simulink model "Variable_Mass_Station_Keeping"  (R2017b)
settings: Solver=VariableStepAuto  StartTime=0.0  StopTime=100  RelTol=1e-3
values from neighbouring files (symbols this model uses):
  A_define = A(1:12,1:12)    [F16_init.m]
  A_la_define = A_define([2,4,6,9,10,12],[2,4,6,9,10,12])    [Controller_para.m]
  A_lon_define = A_define([1,3,5,7,8,11],[1,3,5,7,8,11])    [Controller_para.m]
  airSpeed = 393.720000000000    (= 393.72)    [F16_init.m]
  alpha0 = trimAlpha*180/pi    (= 6.62393794015)    [F16_init.m]
  altitude = 9843    [F16_init.m]
  B_define = A(1:12,13:16)    [F16_init.m]
  B_la_define = B_define([2,4,6,9,10,12],3:4)    [Controller_para.m]
  B_lon_define = B_define([1,3,5,7,8,11],1:2)    [Controller_para.m]
  b_ref = 30.0    (= 30)    [F16_init.m]
  C_la = [1,0,zeros(1,4)]    [F16_init.m]
  C_lon = [1,0,zeros(1,4);0,1,zeros(1,4)]    [F16_init.m]
  CC_la = P_la * B_la_define    [Controller_para.m]
  CC_lon = P_lon * B_lon_define    [Controller_para.m]
  dLEF = 0    [F16_init.m]
  fi_flag = 1    [F16_init.m]
  Inertia = [9496,0,-982.0;0,55814.0,0;-982.0,0,63100.0]    [F16_init.m]
  Ki_la = -k_la(:,9)    [F16_init.m]
  Ki_lon = -k_lon(:,9:10)    [F16_init.m]
  kp_la = Kp_define(3:4,[2,4,6,9,10,12])    [Controller_para.m]    (also in F16_init.m)
  kp_lon = Kp_define(1:2,[1,3,5,7,8,11])    [Controller_para.m]    (also in F16_init.m)
  mass = 636.94    [F16_init.m]
  trim_ail = 0.00874607850103852    (= 0.00874607850104)    [F16_init.m]
  trim_control = [trim_thrust;trim_ele;trim_ail;trim_rud]    [F16_init.m]
  trim_ele = -2.97973164860638    (= -2.97973164861)    [F16_init.m]
  trim_rud = 0.0680302158182712    (= 0.0680302158183)    [F16_init.m]
  trim_state = [0;0;0;0;trimAlpha;0;airSpeed;trimAlpha;0;0;0;0]    [F16_init.m]
  trim_thrust = 2279.08519954656    (= 2279.08519955)    [F16_init.m]
  v_oil = 1.37    [F16_init.m]
undefined symbols (not defined in the file or in its folder): F, MIL
libraries: aerolibasang x8, aerolibconvert2 x8, aerolibobsolete x3, aerolibatmos2 x2, aerolibadyn x2, aerolibwind2 x1, shared6dof x1
(part 2 of 2)

== matlab function Variable_Mass_Station_Keeping/Constant Mass Model/Observer/Nonlinear Term ==
  data: trimed_states input; y output; A_la_define input; A_lon_define input; trim_states input
function y = fcn(trimed_states,A_la_define,A_lon_define,trim_states)
%% 原状态值（配平前的）
ori_states = trimed_states + trim_states;
phi_ori = ori_states(4);
theta_ori = ori_states(5);
psi_ori = ori_states(6);
Vr_ori = ori_states(7);
alpha_ori = ori_states(8);
beta_ori = ori_states(9);
p_ori = ori_states(10);
q_ori = ori_states(11);
r_ori = ori_states(12);

ug_ori = Vr_ori * cos(alpha_ori) * cos(beta_ori);
vg_ori = Vr_ori * sin(beta_ori);
wg_ori = Vr_ori * sin(alpha_ori) * cos(beta_ori);

xg_ori = ug_ori*cos(theta_ori)*cos(psi_ori) + vg_ori*(sin(phi_ori)*sin(theta_ori)*cos(psi_ori)-cos(phi_ori)*sin(psi_ori)) ...
     + wg_ori*(sin(phi_ori)*sin(psi_ori)+cos(phi_ori)*sin(theta_ori)*cos(psi_ori));
yg_ori = ug_ori*cos(theta_ori)*sin(psi_ori) + vg_ori*(sin(phi_ori)*sin(theta_ori)*sin(psi_ori)+cos(phi_ori)*cos(psi_ori)) ...
     + wg_ori*(-sin(phi_ori)*cos(psi_ori) + cos(phi_ori)*sin(theta_ori)*sin(psi_ori));
hg_ori = ug_ori*sin(theta_ori) - vg_ori*sin(phi_ori)*cos(theta_ori) - wg_ori*cos(phi_ori)*cos(theta_ori);
%% 差状态值（配平后的）
phi_trimed = trimed_states(4);
theta_trimed = trimed_states(5);
psi_trimed = trimed_states(6);
Vr_trimed = trimed_states(7);
alpha_trimed = trimed_states(8);
beta_trimed = trimed_states(9);
p_trimed = trimed_states(10);
q_trimed = trimed_states(11);
r_trimed = trimed_states(12);

% x_nonlinear = Vr_ori * cos(theta_ori - alpha_ori) - A_lon_define(1,3) * theta_trimed - Vr_ori;
% y_nonlinear = Vr_ori * cos(theta_ori - alpha_ori) * sin(psi_ori + beta_ori) - A_la_define(1,2) * phi_trimed - A_la_define(1,3) * psi_trimed - A_la_define(1,4) * beta_trimed;
% h_nonlinear = hg_ori  - A_lon_define(2,3) * (theta_trimed - alpha_trimed);

x_nonlinear = Vr_ori * cos(theta_ori - alpha_ori) - trim_states(7)*cos(trim_states(5)-trim_states(8)) - A_lon_define(1,3) * theta_trimed - Vr_trimed;
y_nonlinear = yg_ori - A_la_define(1,2) * phi_trimed - A_la_define(1,3) * psi_trimed - A_la_define(1,4) * beta_trimed;
h_nonlinear = Vr_ori * sin(theta_ori - alpha_ori) - A_lon_define(2,3) * (theta_trimed - alpha_trimed);
psi_nonlinear = (q_ori*sin(phi_ori) + r_ori*cos(phi_ori))/cos(theta_ori) - A_la_define(3,6) * r_trimed;  % psi
phi_nonlinear = p_ori + tan(theta_ori)*(q_ori*sin(phi_ori)+r_ori*cos(phi_ori)) - A_la_define(2,5) * p_trimed - A_la_define(2,6) * r_trimed;  % phi


y = [x_nonlinear; y_nonlinear; h_nonlinear; phi_nonlinear; 0; psi_nonlinear; 0;0;0;0;0;0];

== matlab function Variable_Mass_Station_Keeping/Constant Mass Model/pri_sys_controller/MATLAB Function ==
  settings: updateMethod=DISCRETE
  data: y output; t input
function y = fcn(t)

persistent tt;
if(isempty(tt))
  tt=0;
end

t1 = t-tt;
% if t1 < 10
%     xx = 0;
% elseif  t1 >= 10 && t1 < 70
%     xx = 50*sin(0.025*(t1-10));
% elseif  t1 >= 70 && t1 < 90
%     xx = 50;
% elseif  t1 >= 90 && t1 < 150
%     xx = 50-15*sin(0.025*(t1-90));
% else
%     xx = 35;
% end

% if t1 < 10
%     xx = 0;
% elseif  t1 >= 10 && t1 < 70
%     xx = 1*sin(0.025*(t1-10));
% else
%     xx = 1;
% end
xx = 0;

zz = 0;

y = [xx;zz];

end

== matlab function Variable_Mass_Station_Keeping/Variable Mass Model/sec_sys_controller/Lon_Controller ==
  data: s output; Sec_States input; output output; Pri_States input; A_lon_define input; B_lon_define input; CC_lon input; trim_states input
function [s,output] = Lon_Controller(Sec_States,Pri_States,A_lon_define,B_lon_define,CC_lon,trim_states)
Sec_lon = Sec_States([1,3,5,7,8,11]);  % 辅系统纵向通道状态
ori_states = Sec_States + Pri_States + trim_states;
theta_ori = ori_states(5);
Vr_ori = ori_states(7);
alpha_ori = ori_states(8);

trimed_states = Sec_States + Pri_States;
theta_trimed = trimed_states(5);
Vr_trimed = trimed_states(7);
alpha_trimed = trimed_states(8);

%%  辅系统非线性项g(x)
first_term = Vr_ori * cos(theta_ori - alpha_ori)  - trim_states(7)*cos(trim_states(5)-trim_states(8)) -  A_lon_define(1,3) * theta_trimed - Vr_trimed;
second_term = Vr_ori * sin(theta_ori - alpha_ori) - A_lon_define(2,3) * (theta_trimed - alpha_trimed);
NonLinear = [first_term;second_term;0;0;0;0];
% NonLinear = 0;
%% 滑模控制器结构
s = CC_lon' * Sec_lon;    % 定义滑模面
gain_lon = inv(CC_lon'*B_lon_define);
k1 = [1,0;0,1];
temp = CC_lon'* (A_lon_define * Sec_lon + NonLinear) + k1 * s;
output = -gain_lon * temp;
%% 反馈线性化控制器结构
% s = CC_lon' * Sec_lon;    % 定义输出函数 y = C * x
% gain_lon = inv(CC_lon'*B_lon_define);
% output = gain_lon * (-s - CC_lon' * NonLinear - CC_lon' * A_lon_define * Sec_lon);
end

== matlab function Variable_Mass_Station_Keeping/Variable Mass Model/sec_sys_controller/Lat_Controller ==
  data: Pri_States input; Sec_States input; output output; A_la_define input; B_la_define input; CC_la input; s output; trim_states input
function [output,s] = Lat_Controller(Pri_States,Sec_States,A_la_define,B_la_define,CC_la,trim_states)
Sec_lat = Sec_States([2,4,6,9,10,12]);  % 辅系统横侧向通道状态
ori_states = Sec_States + Pri_States + trim_states;
phi_ori = ori_states(4);
theta_ori = ori_states(5);
psi_ori = ori_states(6);
Vr_ori = ori_states(7);
alpha_ori = ori_states(8);
beta_ori = ori_states(9);
p_ori = ori_states(10);
q_ori = ori_states(11);
r_ori = ori_states(12);

ug_ori = Vr_ori * cos(alpha_ori) * cos(beta_ori);
vg_ori = Vr_ori * sin(beta_ori);
wg_ori = Vr_ori * sin(alpha_ori) * cos(beta_ori);

yg_ori = ug_ori*cos(theta_ori)*sin(psi_ori) + vg_ori*(sin(phi_ori)*sin(theta_ori)*sin(psi_ori)+cos(phi_ori)*cos(psi_ori)) ...
     + wg_ori*(-sin(phi_ori)*cos(psi_ori)+cos(phi_ori)*sin(theta_ori)*sin(psi_ori));
 
trimed_states = Sec_States + Pri_States;
phi_trimed = trimed_states(4);
theta_trimed = trimed_states(5);
psi_trimed = trimed_states(6);
Vr_trimed = trimed_states(7);
alpha_trimed = trimed_states(8);
beta_trimed = trimed_states(9);
p_trimed = trimed_states(10);
q_trimed = trimed_states(11);
r_trimed = trimed_states(12);
%%  辅系统非线性项g(x)
first_term = yg_ori - A_la_define(1,2) * phi_trimed - A_la_define(1,3) * psi_trimed - A_la_define(1,4) * beta_trimed;
% first_term = Vr_ori * cos(theta_ori - alpha_ori) * sin(psi_ori + beta_ori) - A_la_define(1,2) * phi_trimed - A_la_define(1,3) * psi_trimed - A_la_define(1,4) * beta_trimed;
second_term = p_ori + tan(theta_ori)*(q_ori*sin(phi_ori)+r_ori*cos(phi_ori)) - A_la_define(2,5) * p_trimed - A_la_define(2,6) * r_trimed;  % phi
third_term = (q_ori*sin(phi_ori) + r_ori*cos(phi_ori))/cos(theta_ori) - A_la_define(3,6) * r_trimed;  % psi
NonLinear = [first_term;second_term;third_term;0;0;0];
% NonLinear = 0;
%% 滑模控制器结构
s = CC_la' * Sec_lat;    % 定义滑模面
gain_lat = inv(CC_la'*B_la_define);
k1 = [1,0;0,1];
temp = CC_la'* (A_la_define * Sec_lat + NonLinear) + k1 * s ;
output = -gain_lat * temp;
%% 反馈线性化控制器结构
% s = CC_la' * Sec_lat;    % 定义输出函数 y = C * x
% gain_lat = inv(CC_la'*B_la_define);
% output = gain_lat * (-s - CC_la' * NonLinear - CC_la' * A_la_define * Sec_lat);
end

== matlab function Variable_Mass_Station_Keeping/Constant Mass Model/pri_sys_controller/MATLAB Function1 ==
  settings: updateMethod=DISCRETE
  data: y output; t input
function y = fcn(t)

persistent tt;
if(isempty(tt))
  tt=0;
end

t1 = t-tt;

% if t1 < 90
%     yy = 0;
% elseif  t1 >= 90 && t1 < 150
%     yy = 50*sin(0.025*(t1-90));
% else
%     yy = 50;
% end
% end

yy = 0;
y = yy;

== matlab function Variable_Mass_Station_Keeping/Constant Mass Model/pri_sys_controller/MATLAB Function3 ==
  data: u input; y output
function y = fcn(u)

y = u([1,3,5,7,8,11]);

== matlab function Variable_Mass_Station_Keeping/Variable Mass Model/pri_sys_controller/MATLAB Function1 ==
  settings: updateMethod=DISCRETE
  data: y output; t input
function y = fcn(t)

persistent tt;
if(isempty(tt))
  tt=0;
end

t1 = t-tt;

% if t1 < 90
%     yy = 0;
% elseif  t1 >= 90 && t1 < 150
%     yy = 50*sin(0.025*(t1-90));
% else
%     yy = 50;
% end

yy = 0;

y = yy;

end

== matlab function Variable_Mass_Station_Keeping/Variable Mass Model/Observer/Nonlinear Term ==
  data: trimed_states input; y output; A_la_define input; A_lon_define input; trim_states input
function y = fcn(trimed_states,A_la_define,A_lon_define,trim_states)
%% 原状态值（配平前的）
ori_states = trimed_states + trim_states;
phi_ori = ori_states(4);
theta_ori = ori_states(5);
psi_ori = ori_states(6);
Vr_ori = ori_states(7);
alpha_ori = ori_states(8);
beta_ori = ori_states(9);
p_ori = ori_states(10);
q_ori = ori_states(11);
r_ori = ori_states(12);

ug_ori = Vr_ori * cos(alpha_ori) * cos(beta_ori);
vg_ori = Vr_ori * sin(beta_ori);
wg_ori = Vr_ori * sin(alpha_ori) * cos(beta_ori);

xg_ori = ug_ori*cos(theta_ori)*cos(psi_ori) + vg_ori*(sin(phi_ori)*sin(theta_ori)*cos(psi_ori)-cos(phi_ori)*sin(psi_ori)) ...
     + wg_ori*(sin(phi_ori)*sin(psi_ori)+cos(phi_ori)*sin(theta_ori)*cos(psi_ori));
yg_ori = ug_ori*cos(theta_ori)*sin(psi_ori) + vg_ori*(sin(phi_ori)*sin(theta_ori)*sin(psi_ori)+cos(phi_ori)*cos(psi_ori)) ...
     + wg_ori*(-sin(phi_ori)*cos(psi_ori) + cos(phi_ori)*sin(theta_ori)*sin(psi_ori));
hg_ori = ug_ori*sin(theta_ori) - vg_ori*sin(phi_ori)*cos(theta_ori) - wg_ori*cos(phi_ori)*cos(theta_ori);
%% 差状态值（配平后的）
phi_trimed = trimed_states(4);
theta_trimed = trimed_states(5);
psi_trimed = trimed_states(6);
Vr_trimed = trimed_states(7);
alpha_trimed = trimed_states(8);
beta_trimed = trimed_states(9);
p_trimed = trimed_states(10);
q_trimed = trimed_states(11);
r_trimed = trimed_states(12);

% x_nonlinear = Vr_ori * cos(theta_ori - alpha_ori) - A_lon_define(1,3) * theta_trimed - Vr_ori;
% y_nonlinear = Vr_ori * cos(theta_ori - alpha_ori) * sin(psi_ori + beta_ori) - A_la_define(1,2) * phi_trimed - A_la_define(1,3) * psi_trimed - A_la_define(1,4) * beta_trimed;
% h_nonlinear = hg_ori  - A_lon_define(2,3) * (theta_trimed - alpha_trimed);

x_nonlinear = Vr_ori * cos(theta_ori - alpha_ori) - trim_states(7)*cos(trim_states(5)-trim_states(8)) - A_lon_define(1,3) * theta_trimed - Vr_trimed;
y_nonlinear = yg_ori - A_la_define(1,2) * phi_trimed - A_la_define(1,3) * psi_trimed - A_la_define(1,4) * beta_trimed;
h_nonlinear = Vr_ori * sin(theta_ori - alpha_ori) - A_lon_define(2,3) * (theta_trimed - alpha_trimed);
psi_nonlinear = (q_ori*sin(phi_ori) + r_ori*cos(phi_ori))/cos(theta_ori) - A_la_define(3,6) * r_trimed;  % psi
phi_nonlinear = p_ori + tan(theta_ori)*(q_ori*sin(phi_ori)+r_ori*cos(phi_ori)) - A_la_define(2,5) * p_trimed - A_la_define(2,6) * r_trimed;  % phi


y = [x_nonlinear; y_nonlinear; h_nonlinear; phi_nonlinear; 0; psi_nonlinear; 0;0;0;0;0;0];

== matlab function Variable_Mass_Station_Keeping/Constant Mass Model/pri_sys_controller/MATLAB Function4 ==
  data: u input; y output
function y = fcn(u)

y = u([2,4,6,9,10,12]);

== matlab function Variable_Mass_Station_Keeping/Variable Mass Model/pri_sys_controller/MATLAB Function3 ==
  data: u input; y output
function y = fcn(u)

y = u([1,3,5,7,8,11]);

== matlab function Variable_Mass_Station_Keeping/Variable Mass Model/pri_sys_controller/MATLAB Function4 ==
  data: u input; y output
function y = fcn(u)

y = u([2,4,6,9,10,12]);

== matlab function Variable_Mass_Station_Keeping/Constant Mass Model/sec_sys_controller/Lat_Controller ==
  data: Pri_States input; Sec_States input; output output; A_la_define input; B_la_define input; CC_la input; s output; trim_states input
function [output,s] = Lat_Controller(Pri_States,Sec_States,A_la_define,B_la_define,CC_la,trim_states)
Sec_lat = Sec_States([2,4,6,9,10,12]);  % 辅系统横侧向通道状态
ori_states = Sec_States + Pri_States + trim_states;
phi_ori = ori_states(4);
theta_ori = ori_states(5);
psi_ori = ori_states(6);
Vr_ori = ori_states(7);
alpha_ori = ori_states(8);
beta_ori = ori_states(9);
p_ori = ori_states(10);
q_ori = ori_states(11);
r_ori = ori_states(12);

ug_ori = Vr_ori * cos(alpha_ori) * cos(beta_ori);
vg_ori = Vr_ori * sin(beta_ori);
wg_ori = Vr_ori * sin(alpha_ori) * cos(beta_ori);

yg_ori = ug_ori*cos(theta_ori)*sin(psi_ori) + vg_ori*(sin(phi_ori)*sin(theta_ori)*sin(psi_ori)+cos(phi_ori)*cos(psi_ori)) ...
     + wg_ori*(-sin(phi_ori)*cos(psi_ori)+cos(phi_ori)*sin(theta_ori)*sin(psi_ori));
 
trimed_states = Sec_States + Pri_States;
phi_trimed = trimed_states(4);
theta_trimed = trimed_states(5);
psi_trimed = trimed_states(6);
Vr_trimed = trimed_states(7);
alpha_trimed = trimed_states(8);
beta_trimed = trimed_states(9);
p_trimed = trimed_states(10);
q_trimed = trimed_states(11);
r_trimed = trimed_states(12);
%%  辅系统非线性项g(x)
first_term = yg_ori - A_la_define(1,2) * phi_trimed - A_la_define(1,3) * psi_trimed - A_la_define(1,4) * beta_trimed;
% first_term = Vr_ori * cos(theta_ori - alpha_ori) * sin(psi_ori + beta_ori) - A_la_define(1,2) * phi_trimed - A_la_define(1,3) * psi_trimed - A_la_define(1,4) * beta_trimed;
second_term = p_ori + tan(theta_ori)*(q_ori*sin(phi_ori)+r_ori*cos(phi_ori)) - A_la_define(2,5) * p_trimed - A_la_define(2,6) * r_trimed;  % phi
third_term = (q_ori*sin(phi_ori) + r_ori*cos(phi_ori))/cos(theta_ori) - A_la_define(3,6) * r_trimed;  % psi
NonLinear = [first_term;second_term;third_term;0;0;0];
% NonLinear = 0;
%% 滑模控制器结构
s = CC_la' * Sec_lat;    % 定义滑模面
gain_lat = inv(CC_la'*B_la_define);
k1 = [1,0;0,1];
temp = CC_la'* (A_la_define * Sec_lat + NonLinear) + k1 * s ;
output = -gain_lat * temp;
%% 反馈线性化控制器结构
% s = CC_la' * Sec_lat;    % 定义输出函数 y = C * x
% gain_lat = inv(CC_la'*B_la_define);
% output = gain_lat * (-s - CC_la' * NonLinear - CC_la' * A_la_define * Sec_lat);
end

== matlab function Variable_Mass_Station_Keeping/Constant Mass Model/sec_sys_controller/Lon_Controller ==
  data: s output; Sec_States input; output output; Pri_States input; A_lon_define input; B_lon_define input; CC_lon input; trim_states input
function [s,output] = Lon_Controller(Sec_States,Pri_States,A_lon_define,B_lon_define,CC_lon,trim_states)
Sec_lon = Sec_States([1,3,5,7,8,11]);  % 辅系统纵向通道状态
ori_states = Sec_States + Pri_States + trim_states;
theta_ori = ori_states(5);
Vr_ori = ori_states(7);
alpha_ori = ori_states(8);

trimed_states = Sec_States + Pri_States;
theta_trimed = trimed_states(5);
Vr_trimed = trimed_states(7);
alpha_trimed = trimed_states(8);

%%  辅系统非线性项g(x)
first_term = Vr_ori * cos(theta_ori - alpha_ori)  - trim_states(7)*cos(trim_states(5)-trim_states(8)) -  A_lon_define(1,3) * theta_trimed - Vr_trimed;
second_term = Vr_ori * sin(theta_ori - alpha_ori) - A_lon_define(2,3) * (theta_trimed - alpha_trimed);
NonLinear = [first_term;second_term;0;0;0;0];
% NonLinear = 0;
%% 滑模控制器结构
s = CC_lon' * Sec_lon;    % 定义滑模面
gain_lon = inv(CC_lon'*B_lon_define);
k1 = [1,0;0,1];
temp = CC_lon'* (A_lon_define * Sec_lon + NonLinear) + k1 * s;
output = -gain_lon * temp;
%% 反馈线性化控制器结构
% s = CC_lon' * Sec_lon;    % 定义输出函数 y = C * x
% gain_lon = inv(CC_lon'*B_lon_define);
% output = gain_lon * (-s - CC_lon' * NonLinear - CC_lon' * A_lon_define * Sec_lon);
end
